simulink model "example_simulink"  (R2024a)
settings: Solver=VariableStepAuto  StartTime=0.0  StopTime=10.0  RelTol=1e-3
values from neighbouring files (symbols this model uses):
  A = double(A)    [get_k_length.m]
  B = double(B)    [get_k_length.m]
  K = lqr(A,B,Q,R)    [get_k_length.m]
  L0 = sqrt(L2^2 - (L5/2 - L1 .* cos(phi1_rad)).^2) + L1 .* sin(phi1_rad)    [leg_calculate.m]
undefined symbols (not defined in the file or in its folder): Ld, zd, zf
libraries: slpidlib x1
settings Model: Creator=lenovo  LastModifiedBy=lenovo
settings DebuggingCC: UnconnectedInputMsg=warning  UnconnectedOutputMsg=warning  UnconnectedLineMsg=warning
settings ModelReferenceCC: EnableRefExpFcnMdlSchedulingChecks=on
settings RTWCC: GPUComputeCapability=3.5  DLArmComputeVersion=19.05

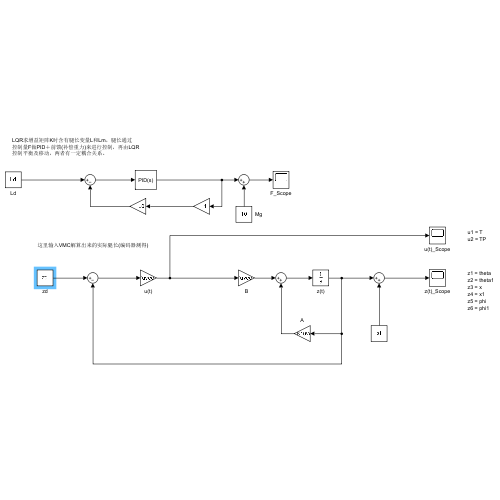
[thumbnail: Simulink's stored preview of the top-level diagram]
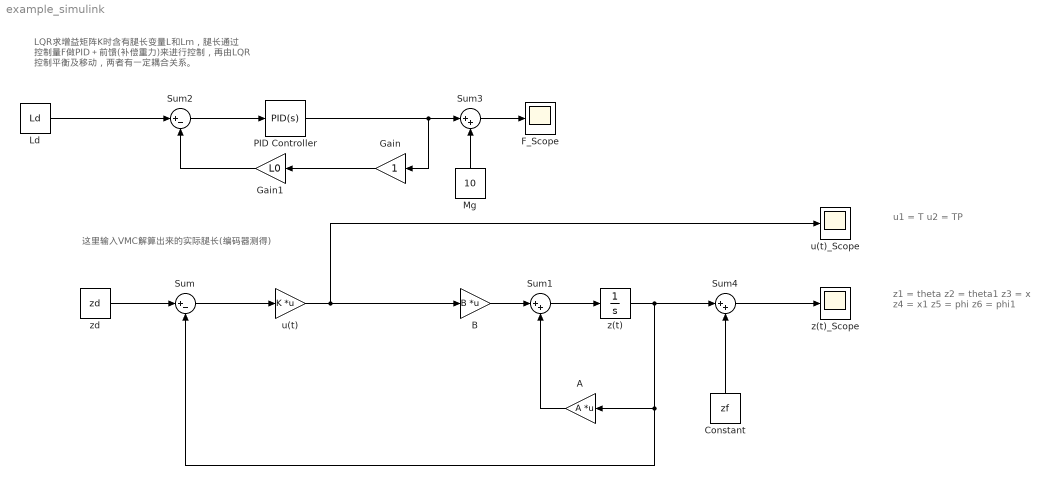
== system example_simulink ==
  note: 这里输入VMC解算出来的实际腿长(编码器测得)
  note: LQR求增益矩阵K时含有腿长变量L和Lm，腿长通过
      | 控制量F做PID＋前馈(补偿重力)来进行控制，再由LQR
      | 控制平衡及移动，两者有一定耦合关系。
  note: z1 = theta
      | z2 = theta1
      | z3 = x
      | z4 = x1
      | z5 = phi
      | z6 = phi1
  note: u1 = T
      | u2 = TP
  A : Gain  Gain=A  Multiplication=Matrix(K*u) (u vector)
  B : Gain  Gain=B  Multiplication=Matrix(K*u) (u vector)
  Constant : Constant  Value=zf
  F_Scope : Scope
  Gain : Gain
  Gain1 : Gain  Gain=L0
  Ld : Constant  Value=Ld
  Mg : Constant  Value=10
  PID Controller : slpidlib/PID Controller  Controller=PID  Form=Parallel  TimeDomain=Continuous-time  UseExternalTs=off  SampleTime=-1  IntegratorMethod=Forward Euler  FilterMethod=Forward Euler  ControllerParametersSource=internal  P=10  I=0.01  UseKiTs=off  D=0  UseExternalDerivativeSource=off  N=100  UseFilter=on  TunerSelectOption=Transfer Function Based (PID Tuner App)  InitialConditionSource=internal  InitialConditionForIntegrator=0  InitialConditionForFilter=0  DifferentiatorICPrevScaledInput=0  ExternalReset=none  TrackingMode=off  Kt=1  LimitOutput=off  SatLimitsSource=internal  UpperSaturationLimit=inf  LowerSaturationLimit=-inf  LinearizeAsGain=on  AntiWindupMode=none  Kb=1  LimitIntegrator=off  UpperIntegratorSaturationLimit=inf  LowerIntegratorSaturationLimit=-inf  POutMin=[]  POutMax=[]  IOutMin=[]  IOutMax=[]  DOutMin=[]  DOutMax=[]  NOutMin=[]  NOutMax=[]  SumOutMin=[]  SumOutMax=[]  SaturationOutMin=[]  SaturationOutMax=[]  PParamMin=[]  PParamMax=[]  IParamMin=[]  IParamMax=[]  DParamMin=[]  DParamMax=[]  NParamMin=[]  NParamMax=[]  KbParamMin=[]  KbParamMax=[]  KtParamMin=[]  KtParamMax=[]  KbOutMin=[]  KbOutMax=[]  KtOutMin=[]  KtOutMax=[]  IntegratorOutMin=[]  IntegratorOutMax=[]  FilterOutMin=[]  FilterOutMax=[]  SumI1OutMin=[]  SumI1OutMax=[]  SumI2OutMin=[]  SumI2OutMax=[]  SumI3OutMin=[]  SumI3OutMax=[]  SumI4OutMin=[]  SumI4OutMax=[]  SumDOutMin=[]  SumDOutMax=[]  DifferentiatorOutMin=[]  DifferentiatorOutMax=[]  FilterDiffOutCoefMin=[]  FilterDiffOutCoefMax=[]  ReciprocalOutMin=[]  ReciprocalOutMax=[]  SumDenOutMin=[]  SumDenOutMax=[]  SumNumOutMin=[]  SumNumOutMax=[]  DivideOutMin=[]  DivideOutMax=[]  UdiffTsProdOutMin=[]  UdiffTsProdOutMax=[]  NTsProdOutMin=[]  NTsProdOutMax=[]  UintegralTsProdOutMin=[]  UintegralTsProdOutMax=[]  UngainTsProdOutMin=[]  UngainTsProdOutMax=[]  ClampingZeroOutDataTypeStr=Inherit: Inherit via back propagation  ClampingZeroOutMin=[]  ClampingZeroOutMax=[]  FilterDenConstantOutDataTypeStr=Inherit: Inherit via back propagation  FilterDenConstantOutMin=[]  FilterDenConstantOutMax=[]  PCopyOutDataTypeStr=Inherit: Inherit via back propagation  PCopyOutMin=[]  PCopyOutMax=[]  NCopyOutDataTypeStr=Inherit: Inherit via back propagation  NCopyOutMin=[]  NCopyOutMax=[]  IntegratorContinuousStateAttributes=''  IntegratorStateMustResolveToSignalObject=off  IntegratorRTWStateStorageClass=Auto  FilterContinuousStateAttributes=''  FilterStateMustResolveToSignalObject=off  FilterRTWStateStorageClass=Auto  ParallelPVariant=InternalParameters  IdealPVariant=Disabled  IVariant=InternalParameters  DVariant=InternalParameters  IntegratorVariant=Continuous  SatVariant=Disabled  AWVariant=Passthrough  PCopyVariant=Disabled  TRVariant=Disabled  FdbkBlocksVariant=Forward  IdealPFdbkVariant=Disabled  SatFdbkVariant=Disabled  DerivativeFilterVariant=ContFilter  NVariant=InternalParameters  NCopyVariant=Disabled  FilterICVariant=InternalICsFilter  IntegratorICVariant=InternalICs  ExternalResetVariant=Disabled  TRSumVariant=Passthrough  SumFdbkVariant=Disabled  SumVariant=Sum_PID  TsampFilterVariant=InternalTs  TsampNgainVariant=Passthrough  TsampIntegralVariant=Disabled_SignalSpec  ExternalSaturationOutDataTypeStr=Inherit: Same as second input  DerivativeSourceVariant=ErrorSignal
  Sum : Sum  Inputs=|+-
  Sum1 : Sum  Inputs=|++
  Sum2 : Sum  Inputs=|+-
  Sum3 : Sum  Inputs=|++
  Sum4 : Sum  Inputs=|++
  u(t) : Gain  Gain=K  Multiplication=Matrix(K*u) (u vector)
  u(t)_Scope : Scope
  z(t) : Integrator
  z(t)_Scope : Scope
  zd : Constant  Value=zd
  wires:
  zd/1 -> Sum/1
  Sum/1 -> u(t)/1
  u(t)/1 -> u(t)_Scope/1, B/1
  B/1 -> Sum1/1
  Sum1/1 -> z(t)/1
  A/1 -> Sum1/2
  z(t)/1 -> Sum4/1, Sum/2, A/1
  Ld/1 -> Sum2/1
  Sum2/1 -> PID Controller/1
  PID Controller/1 -> Sum3/1, Gain/1
  Gain1/1 -> Sum2/2
  Gain/1 -> Gain1/1
  Mg/1 -> Sum3/2
  Sum3/1 -> F_Scope/1
  Sum4/1 -> z(t)_Scope/1
  Constant/1 -> Sum4/2
